simulink model "qdr_vacc_10"  (Simulink 7.9)
settings: Solver=ode45  StartTime=0.0  StopTime=10.0  RelTol=1e-3
libraries: xbsIndex_r4 x8, casper_library_accumulators x1
settings Model: Creator=tfiliba  LastModifiedBy=tfiliba

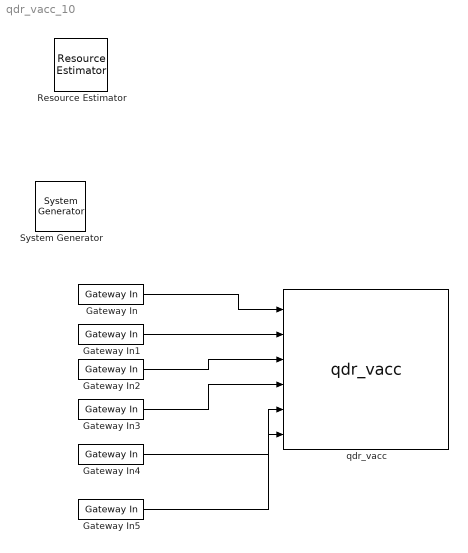
== system qdr_vacc_10 ==
  " System Generator" : xbsIndex_r4/ System Generator  Tag=genX  xilinxfamily=Kintex7  part=xc7k325t  speed=-3  package=fbg676  synthesis_tool=XST  clock_wrapper=Clock Enables  directory=./netlist  proj_type=Project Navigator  Synth_file=XST Defaults  Impl_file=ISE Defaults  testbench=off  simulink_period=1  sysclk_period=10  dcm_input_clock_period=10  incr_netlist=off  trim_vbits=Everywhere in SubSystem  dbl_ovrd=According to Block Masks  core_generation=According to Block Masks  run_coregen=off  deprecated_control=off  eval_field=0  block_type=sysgen
  Gateway In : xbsIndex_r4/Gateway In  gui_display_data_type=Fixed-point  arith_type="Signed  (2's comp)"  n_bits=16  bin_pt=14  preci_type=Single  exp_width=8  frac_width=24  quantization="Round  (unbiased: +/- Inf)"  overflow=Saturate  period=1  dbl_ovrd=off  timing_constraint=None  locs_specified=off  LOCs={}  UseAsADC=off  ADCChannel='1'  inherit_from_input=off  hdl_port=on  block_type=gatewayin
      settings: xl_area=[0 0 0 0 16 0 0]
  Gateway In1 : xbsIndex_r4/Gateway In  gui_display_data_type=Boolean  arith_type=Boolean  n_bits=16  bin_pt=14  preci_type=Single  exp_width=8  frac_width=24  quantization="Round  (unbiased: +/- Inf)"  overflow=Saturate  period=1  dbl_ovrd=off  timing_constraint=None  locs_specified=off  LOCs={}  UseAsADC=off  ADCChannel='1'  inherit_from_input=off  hdl_port=on  block_type=gatewayin
      settings: xl_area=[0 0 0 0 1 0 0]
  Gateway In2 : xbsIndex_r4/Gateway In  gui_display_data_type=Fixed-point  arith_type="Signed  (2's comp)"  n_bits=32  bin_pt=0  preci_type=Single  exp_width=8  frac_width=24  quantization="Round  (unbiased: +/- Inf)"  overflow=Saturate  period=1  dbl_ovrd=off  timing_constraint=None  locs_specified=off  LOCs={}  UseAsADC=off  ADCChannel='1'  inherit_from_input=off  hdl_port=on  block_type=gatewayin
      settings: xl_area=[0 0 0 0 32 0 0]
  Gateway In3 : xbsIndex_r4/Gateway In  gui_display_data_type=Fixed-point  arith_type=Unsigned  n_bits=4  bin_pt=0  preci_type=Single  exp_width=8  frac_width=24  quantization="Round  (unbiased: +/- Inf)"  overflow=Saturate  period=1  dbl_ovrd=off  timing_constraint=None  locs_specified=off  LOCs={}  UseAsADC=off  ADCChannel='1'  inherit_from_input=off  hdl_port=on  block_type=gatewayin
      settings: xl_area=[0 0 0 0 4 0 0]
  Gateway In4 : xbsIndex_r4/Gateway In  gui_display_data_type=Boolean  arith_type=Boolean  n_bits=16  bin_pt=14  preci_type=Single  exp_width=8  frac_width=24  quantization="Round  (unbiased: +/- Inf)"  overflow=Saturate  period=1  dbl_ovrd=off  timing_constraint=None  locs_specified=off  LOCs={}  UseAsADC=off  ADCChannel='1'  inherit_from_input=off  hdl_port=on  block_type=gatewayin
      settings: xl_area=[0 0 0 0 1 0 0]
  Gateway In5 : xbsIndex_r4/Gateway In  gui_display_data_type=Boolean  arith_type=Boolean  n_bits=16  bin_pt=14  preci_type=Single  exp_width=8  frac_width=24  quantization="Round  (unbiased: +/- Inf)"  overflow=Saturate  period=1  dbl_ovrd=off  timing_constraint=None  locs_specified=off  LOCs={}  UseAsADC=off  ADCChannel='1'  inherit_from_input=off  hdl_port=on  block_type=gatewayin
      settings: xl_area=[0 0 0 0 1 0 0]
  Resource Estimator : xbsIndex_r4/Resource Estimator  Tag=resEstTag  Slices=0  FFs=0  BRAMs=0  LUTs=0  IOBs=0  EBMs=0  TBUFs=0  xl_use_estimator_area=off  est_options=Estimate  xl_estimator_area=[824 828 19 1221 232 0 0]  block_type=resource_estimator
      settings: AttributesFormatString=Resource\nEstimator
  qdr_vacc : casper_library_accumulators/qdr_vacc  vector_len=1024
      link override acc_ctrl/rd_addr/convert: arith_type=Unsigned  n_bits=32  bin_pt=0
      link override qdr/convert_be: n_bits=4
      link override qdr/convert_data_in: n_bits=36
      link override qdr/convert_data_in1: n_bits=36
      link override qdr/qdr_latency: latency=10
      link override qdr/qdr_vacc_10_qdr_vacc_qdr_data_out: n_bits=36
      link override status/convert: arith_type=Unsigned  n_bits=32  bin_pt=0
      settings: AttributesFormatString=Vector Length: 1024
      link override Convert1: xl_area=[0 0 0 0 0 0 0]
      link override Delay2: xl_area=[1 1 0 1 0 0 0]
      link override Delay3: xl_area=[1 1 0 1 0 0 0]
      link override Gateway Out1: xl_area=[0 0 0 0 0 0 0]
      link override Gateway Out10: xl_area=[0 0 0 0 0 0 0]
      link override Gateway Out11: xl_area=[0 0 0 0 0 0 0]
      link override Gateway Out12: xl_area=[0 0 0 0 0 0 0]
      link override Gateway Out13: xl_area=[0 0 0 0 0 0 0]
      link override Gateway Out14: xl_area=[0 0 0 0 0 0 0]
      link override Gateway Out15: xl_area=[0 0 0 0 0 0 0]
      link override Gateway Out16: xl_area=[0 0 0 0 0 0 0]
      link override Gateway Out17: xl_area=[0 0 0 0 0 0 0]
      link override Gateway Out18: xl_area=[0 0 0 0 0 0 0]
      link override Gateway Out19: xl_area=[0 0 0 0 0 0 0]
      link override Gateway Out2: xl_area=[0 0 0 0 0 0 0]
      link override Gateway Out20: xl_area=[0 0 0 0 0 0 0]
      link override Gateway Out21: xl_area=[0 0 0 0 0 0 0]
      link override Gateway Out22: xl_area=[0 0 0 0 0 0 0]
      link override Gateway Out23: xl_area=[0 0 0 0 0 0 0]
      link override Gateway Out24: xl_area=[0 0 0 0 0 0 0]
      link override Gateway Out25: xl_area=[0 0 0 0 0 0 0]
      link override Gateway Out26: xl_area=[0 0 0 0 0 0 0]
      link override Gateway Out27: xl_area=[0 0 0 0 0 0 0]
      link override Gateway Out28: xl_area=[0 0 0 0 0 0 0]
      link override Gateway Out29: xl_area=[0 0 0 0 0 0 0]
      link override Gateway Out3: xl_area=[0 0 0 0 0 0 0]
      link override Gateway Out30: xl_area=[0 0 0 0 0 0 0]
      link override Gateway Out31: xl_area=[0 0 0 0 0 0 0]
      link override Gateway Out32: xl_area=[0 0 0 0 0 0 0]
      link override Gateway Out33: xl_area=[0 0 0 0 0 0 0]
      link override Gateway Out4: xl_area=[0 0 0 0 0 0 0]
      link override Gateway Out5: xl_area=[0 0 0 0 0 0 0]
      link override Gateway Out6: xl_area=[0 0 0 0 0 0 0]
      link override Gateway Out7: xl_area=[0 0 0 0 0 0 0]
      link override Gateway Out8: xl_area=[0 0 0 0 0 0 0]
      link override Gateway Out9: xl_area=[0 0 0 0 0 0 0]
      link override Inverter: xl_area=[0 0 0 0 0 0 0]
      link override Inverter1: xl_area=[0 0 0 0 0 0 0]
      link override Logical1: xl_area=[1 1 0 1 0 0 0]
      link override Logical2: xl_area=[1 0 0 1 0 0 0]
      link override Logical3: xl_area=[1 0 0 1 0 0 0]
      link override Logical4: xl_area=[1 0 0 1 0 0 0]
      link override Logical5: xl_area=[1 0 0 1 0 0 0]
      link override Logical6: xl_area=[1 0 0 1 0 0 0]
      link override Relational: xl_area=[6 0 0 11 0 0 0]
      link override Relational1: xl_area=[3 0 0 5 0 0 0]
      link override acc/AddSub4: xl_area=[4 4 0 4 0 0 0]
      link override acc/AddSub5: xl_area=[32 32 0 32 0 0 0]
      link override acc/rd_addr_sel: xl_area=[18 0 0 36 0 0 0]
      link override acc_ctrl/Delay1: xl_area=[1 1 0 0 0 0 0]
      link override acc_ctrl/Delay2: xl_area=[1 1 0 1 0 0 0]
      link override acc_ctrl/Delay3: xl_area=[1 1 0 1 0 0 0]
      link override acc_ctrl/Delay4: xl_area=[5 10 0 0 0 0 0]
      link override acc_ctrl/Delay6: xl_area=[1 1 0 0 0 0 0]
      link override acc_ctrl/Gateway Out1: xl_area=[0 0 0 0 0 0 0]
      link override acc_ctrl/Gateway Out10: xl_area=[0 0 0 0 0 0 0]
      link override acc_ctrl/Gateway Out11: xl_area=[0 0 0 0 0 0 0]
      link override acc_ctrl/Gateway Out12: xl_area=[0 0 0 0 0 0 0]
      link override acc_ctrl/Gateway Out13: xl_area=[0 0 0 0 0 0 0]
      link override acc_ctrl/Gateway Out14: xl_area=[0 0 0 0 0 0 0]
      link override acc_ctrl/Gateway Out15: xl_area=[0 0 0 0 0 0 0]
      link override acc_ctrl/Gateway Out16: xl_area=[0 0 0 0 0 0 0]
      link override acc_ctrl/Gateway Out17: xl_area=[0 0 0 0 0 0 0]
      link override acc_ctrl/Gateway Out19: xl_area=[0 0 0 0 0 0 0]
      link override acc_ctrl/Gateway Out2: xl_area=[0 0 0 0 0 0 0]
      link override acc_ctrl/Gateway Out22: xl_area=[0 0 0 0 0 0 0]
      link override acc_ctrl/Gateway Out28: xl_area=[0 0 0 0 0 0 0]
      link override acc_ctrl/Gateway Out3: xl_area=[0 0 0 0 0 0 0]
      link override acc_ctrl/Gateway Out4: xl_area=[0 0 0 0 0 0 0]
      link override acc_ctrl/Gateway Out5: xl_area=[0 0 0 0 0 0 0]
      link override acc_ctrl/Gateway Out6: xl_area=[0 0 0 0 0 0 0]
      link override acc_ctrl/Gateway Out7: xl_area=[0 0 0 0 0 0 0]
      link override acc_ctrl/Gateway Out8: xl_area=[0 0 0 0 0 0 0]
      link override acc_ctrl/Gateway Out9: xl_area=[0 0 0 0 0 0 0]
      link override acc_ctrl/Inverter: xl_area=[0 0 0 0 0 0 0]
      link override acc_ctrl/Inverter1: xl_area=[0 0 0 0 0 0 0]
      link override acc_ctrl/Inverter2: xl_area=[0 0 0 0 0 0 0]
      link override acc_ctrl/Inverter3: xl_area=[0 0 0 0 0 0 0]
      link override acc_ctrl/Inverter4: xl_area=[0 0 0 0 0 0 0]
      link override acc_ctrl/Inverter5: xl_area=[0 0 0 0 0 0 0]
      link override acc_ctrl/Inverter6: xl_area=[0 0 0 0 0 0 0]
      link override acc_ctrl/Inverter7: xl_area=[0 0 0 0 0 0 0]
      link override acc_ctrl/Inverter8: xl_area=[0 0 0 0 0 0 0]
      link override acc_ctrl/Logical1: xl_area=[1 0 0 1 0 0 0]
      link override acc_ctrl/Logical10: xl_area=[1 0 0 1 0 0 0]
      link override acc_ctrl/Logical11: xl_area=[1 0 0 1 0 0 0]
      link override acc_ctrl/Logical2: xl_area=[1 0 0 1 0 0 0]
      link override acc_ctrl/Logical3: xl_area=[1 0 0 1 0 0 0]
      link override acc_ctrl/Logical4: xl_area=[1 0 0 1 0 0 0]
      link override acc_ctrl/Logical5: xl_area=[1 0 0 1 0 0 0]
      link override acc_ctrl/Logical6: xl_area=[1 0 0 1 0 0 0]
      link override acc_ctrl/Logical7: xl_area=[1 0 0 1 0 0 0]
      link override acc_ctrl/Logical8: xl_area=[1 0 0 1 0 0 0]
      link override acc_ctrl/Logical9: xl_area=[1 0 0 1 0 0 0]
      link override acc_ctrl/Register1: xl_area=[1 1 0 0 0 0 0]
      link override acc_ctrl/Register4: xl_area=[1 1 0 0 0 0 0]
      link override acc_ctrl/Relational: xl_area=[6 0 0 11 0 0 0]
      link override acc_ctrl/Relational2: xl_area=[24 0 0 47 0 0 0]
      link override acc_ctrl/Relational3: xl_area=[6 0 0 11 0 0 0]
      link override acc_ctrl/delay_adder: xl_area=[5 10 0 10 0 0 0]
      link override acc_ctrl/delay_blank_qdr: xl_area=[1 1 0 1 0 0 0]
      link override acc_ctrl/delay_even_addr: xl_area=[5 10 0 0 0 0 0]
      link override acc_ctrl/delay_even_addr1: xl_area=[1 1 0 0 0 0 0]
      link override acc_ctrl/delay_even_addr2: xl_area=[1 1 0 0 0 0 0]
      link override acc_ctrl/delay_for_even_op: xl_area=[1 1 0 0 0 0 0]
      link override acc_ctrl/delay_qdr: xl_area=[5 10 0 10 0 0 0]
      link override acc_ctrl/delay_rd_align: xl_area=[1 1 0 1 0 0 0]
      link override acc_ctrl/delay_rd_align1: xl_area=[1 1 0 1 0 0 0]
      link override acc_ctrl/delay_rd_wr_align1: xl_area=[1 1 0 1 0 0 0]
      link override acc_ctrl/delay_wr_align: xl_area=[5 10 0 10 0 0 0]
      link override acc_ctrl/delay_wr_align1: xl_area=[1 1 0 1 0 0 0]
      link override acc_ctrl/delay_wr_align2: xl_area=[1 1 0 1 0 0 0]
      link override acc_ctrl/delay_wr_align3: xl_area=[1 1 0 1 0 0 0]
      link override acc_ctrl/ease_timing1: xl_area=[8 16 0 0 0 0 0]
      link override acc_ctrl/pulse_ext/Counter3: xl_area=[4 5 0 6 0 0 0]
      link override acc_ctrl/pulse_ext/Gateway Out1: xl_area=[0 0 0 0 0 0 0]
      link override acc_ctrl/pulse_ext/Gateway Out2: xl_area=[0 0 0 0 0 0 0]
      link override acc_ctrl/pulse_ext/Gateway Out3: xl_area=[0 0 0 0 0 0 0]
      link override acc_ctrl/pulse_ext/Gateway Out31: xl_area=[0 0 0 0 0 0 0]
      link override acc_ctrl/pulse_ext/Logical1: xl_area=[1 0 0 1 0 0 0]
      link override acc_ctrl/pulse_ext/Relational5: xl_area=[2 0 0 3 0 0 0]
      link override acc_ctrl/pulse_ext1/Counter3: xl_area=[3 4 0 4 0 0 0]
      link override acc_ctrl/pulse_ext1/Logical: xl_area=[1 0 0 1 0 0 0]
      link override acc_ctrl/pulse_ext1/Logical1: xl_area=[1 0 0 1 0 0 0]
      link override acc_ctrl/pulse_ext1/Register: xl_area=[1 1 0 0 0 0 0]
      link override acc_ctrl/pulse_ext1/Relational5: xl_area=[1 0 0 2 0 0 0]
      link override acc_ctrl/rb_addr: xl_area=[6 10 0 10 0 0 0]
      link override acc_ctrl/rd_addr/convert: xl_area=[0 0 0 0 0 0 0]
      link override acc_ctrl/rd_addr/qdr_vacc_10_qdr_vacc_acc_ctrl_rd_addr_user_data_in: xl_area=[0 0 0 0 32 0 0]
      link override acc_ctrl/rd_addr_cnt: xl_area=[6 10 0 10 0 0 0]
      link override acc_ctrl/rd_addr_sel: xl_area=[5 0 0 10 0 0 0]
      link override acc_ctrl/rd_nwr: xl_area=[5 0 0 10 0 0 0]
      link override acc_ctrl/reg_del: xl_area=[5 10 0 0 0 0 0]
      link override acc_ctrl/vect_cnt: xl_area=[17 32 0 32 0 0 0]
      link override delay: xl_area=[18 36 0 0 0 0 0]
      link override delay1: xl_area=[1 1 0 0 0 0 0]
      link override delay2: xl_area=[1 1 0 0 0 0 0]
      link override fifo_in: xl_area=[29 32 9 50 0 0 0]
      link override fifo_out: xl_area=[29 32 10 50 0 0 0]
      link override make_odd_delay: xl_area=[18 36 0 0 0 0 0]
      link override make_odd_delay1: xl_area=[1 1 0 0 0 0 0]
      link override negedge_delay/Counter3: xl_area=[13 24 0 24 0 0 0]
      link override negedge_delay/Delay: xl_area=[1 1 0 0 0 0 0]
      link override negedge_delay/Logical: xl_area=[1 0 0 1 0 0 0]
      link override negedge_delay/Relational5: xl_area=[13 0 0 25 0 0 0]
      link override negedge_delay/negedge/Delay: xl_area=[1 1 0 0 0 0 0]
      link override negedge_delay/negedge/Inverter: xl_area=[0 0 0 0 0 0 0]
      link override negedge_delay/negedge/Logical: xl_area=[1 0 0 1 0 0 0]
      link override negedge_delay1/Counter3: xl_area=[13 24 0 24 0 0 0]
      link override negedge_delay1/Delay: xl_area=[1 1 0 0 0 0 0]
      link override negedge_delay1/Logical: xl_area=[1 0 0 1 0 0 0]
      link override negedge_delay1/Relational5: xl_area=[13 0 0 25 0 0 0]
      link override negedge_delay1/negedge/Delay: xl_area=[1 1 0 0 0 0 0]
      link override negedge_delay1/negedge/Inverter: xl_area=[0 0 0 0 0 0 0]
      link override negedge_delay1/negedge/Logical: xl_area=[1 0 0 1 0 0 0]
      link override negedge_delay10/Counter3: xl_area=[13 24 0 24 0 0 0]
      link override negedge_delay10/Delay: xl_area=[1 1 0 0 0 0 0]
      link override negedge_delay10/Logical: xl_area=[1 0 0 1 0 0 0]
      link override negedge_delay10/Relational5: xl_area=[13 0 0 25 0 0 0]
      link override negedge_delay10/negedge/Delay: xl_area=[1 1 0 0 0 0 0]
      link override negedge_delay10/negedge/Inverter: xl_area=[0 0 0 0 0 0 0]
      link override negedge_delay10/negedge/Logical: xl_area=[1 0 0 1 0 0 0]
      link override negedge_delay11/Counter3: xl_area=[13 24 0 24 0 0 0]
      link override negedge_delay11/Delay: xl_area=[1 1 0 0 0 0 0]
      link override negedge_delay11/Logical: xl_area=[1 0 0 1 0 0 0]
      link override negedge_delay11/Relational5: xl_area=[13 0 0 25 0 0 0]
      link override negedge_delay11/negedge/Delay: xl_area=[1 1 0 0 0 0 0]
      link override negedge_delay11/negedge/Inverter: xl_area=[0 0 0 0 0 0 0]
      link override negedge_delay11/negedge/Logical: xl_area=[1 0 0 1 0 0 0]
      link override negedge_delay12/Counter3: xl_area=[13 24 0 24 0 0 0]
      link override negedge_delay12/Delay: xl_area=[1 1 0 0 0 0 0]
      link override negedge_delay12/Logical: xl_area=[1 0 0 1 0 0 0]
      link override negedge_delay12/Relational5: xl_area=[13 0 0 25 0 0 0]
      link override negedge_delay12/negedge/Delay: xl_area=[1 1 0 0 0 0 0]
      link override negedge_delay12/negedge/Inverter: xl_area=[0 0 0 0 0 0 0]
      link override negedge_delay12/negedge/Logical: xl_area=[1 0 0 1 0 0 0]
      link override negedge_delay13/Counter3: xl_area=[13 24 0 24 0 0 0]
      link override negedge_delay13/Delay: xl_area=[1 1 0 0 0 0 0]
      link override negedge_delay13/Logical: xl_area=[1 0 0 1 0 0 0]
      link override negedge_delay13/Relational5: xl_area=[13 0 0 25 0 0 0]
      link override negedge_delay13/negedge/Delay: xl_area=[1 1 0 0 0 0 0]
      link override negedge_delay13/negedge/Inverter: xl_area=[0 0 0 0 0 0 0]
      link override negedge_delay13/negedge/Logical: xl_area=[1 0 0 1 0 0 0]
      link override negedge_delay2/Counter3: xl_area=[13 24 0 24 0 0 0]
      link override negedge_delay2/Delay: xl_area=[1 1 0 0 0 0 0]
      link override negedge_delay2/Logical: xl_area=[1 0 0 1 0 0 0]
      link override negedge_delay2/Relational5: xl_area=[13 0 0 25 0 0 0]
      link override negedge_delay2/negedge/Delay: xl_area=[1 1 0 0 0 0 0]
      link override negedge_delay2/negedge/Inverter: xl_area=[0 0 0 0 0 0 0]
      link override negedge_delay2/negedge/Logical: xl_area=[1 0 0 1 0 0 0]
      link override negedge_delay3/Counter3: xl_area=[13 24 0 24 0 0 0]
      link override negedge_delay3/Delay: xl_area=[1 1 0 0 0 0 0]
      link override negedge_delay3/Logical: xl_area=[1 0 0 1 0 0 0]
      link override negedge_delay3/Relational5: xl_area=[13 0 0 25 0 0 0]
      link override negedge_delay3/negedge/Delay: xl_area=[1 1 0 0 0 0 0]
      link override negedge_delay3/negedge/Inverter: xl_area=[0 0 0 0 0 0 0]
      link override negedge_delay3/negedge/Logical: xl_area=[1 0 0 1 0 0 0]
      link override negedge_delay4/Counter3: xl_area=[13 24 0 24 0 0 0]
      link override negedge_delay4/Delay: xl_area=[1 1 0 0 0 0 0]
      link override negedge_delay4/Logical: xl_area=[1 0 0 1 0 0 0]
      link override negedge_delay4/Relational5: xl_area=[13 0 0 25 0 0 0]
      link override negedge_delay4/negedge/Delay: xl_area=[1 1 0 0 0 0 0]
      link override negedge_delay4/negedge/Inverter: xl_area=[0 0 0 0 0 0 0]
      link override negedge_delay4/negedge/Logical: xl_area=[1 0 0 1 0 0 0]
      link override negedge_delay5/Counter3: xl_area=[13 24 0 24 0 0 0]
      link override negedge_delay5/Delay: xl_area=[1 1 0 0 0 0 0]
      link override negedge_delay5/Logical: xl_area=[1 0 0 1 0 0 0]
      link override negedge_delay5/Relational5: xl_area=[13 0 0 25 0 0 0]
      link override negedge_delay5/negedge/Delay: xl_area=[1 1 0 0 0 0 0]
      link override negedge_delay5/negedge/Inverter: xl_area=[0 0 0 0 0 0 0]
      link override negedge_delay5/negedge/Logical: xl_area=[1 0 0 1 0 0 0]
      link override negedge_delay6/Counter3: xl_area=[13 24 0 24 0 0 0]
      link override negedge_delay6/Delay: xl_area=[1 1 0 0 0 0 0]
      link override negedge_delay6/Logical: xl_area=[1 0 0 1 0 0 0]
      link override negedge_delay6/Relational5: xl_area=[13 0 0 25 0 0 0]
      link override negedge_delay6/negedge/Delay: xl_area=[1 1 0 0 0 0 0]
      link override negedge_delay6/negedge/Inverter: xl_area=[0 0 0 0 0 0 0]
      link override negedge_delay6/negedge/Logical: xl_area=[1 0 0 1 0 0 0]
      link override negedge_delay7/Counter3: xl_area=[13 24 0 24 0 0 0]
      link override negedge_delay7/Delay: xl_area=[1 1 0 0 0 0 0]
      link override negedge_delay7/Logical: xl_area=[1 0 0 1 0 0 0]
      link override negedge_delay7/Relational5: xl_area=[13 0 0 25 0 0 0]
      link override negedge_delay7/negedge/Delay: xl_area=[1 1 0 0 0 0 0]
      link override negedge_delay7/negedge/Inverter: xl_area=[0 0 0 0 0 0 0]
      link override negedge_delay7/negedge/Logical: xl_area=[1 0 0 1 0 0 0]
      link override negedge_delay8/Counter3: xl_area=[13 24 0 24 0 0 0]
      link override negedge_delay8/Delay: xl_area=[1 1 0 0 0 0 0]
      link override negedge_delay8/Logical: xl_area=[1 0 0 1 0 0 0]
      link override negedge_delay8/Relational5: xl_area=[13 0 0 25 0 0 0]
      link override negedge_delay8/negedge/Delay: xl_area=[1 1 0 0 0 0 0]
      link override negedge_delay8/negedge/Inverter: xl_area=[0 0 0 0 0 0 0]
      link override negedge_delay8/negedge/Logical: xl_area=[1 0 0 1 0 0 0]
      link override negedge_delay9/Counter3: xl_area=[13 24 0 24 0 0 0]
      link override negedge_delay9/Delay: xl_area=[1 1 0 0 0 0 0]
      link override negedge_delay9/Logical: xl_area=[1 0 0 1 0 0 0]
      link override negedge_delay9/Relational5: xl_area=[13 0 0 25 0 0 0]
      link override negedge_delay9/negedge/Delay: xl_area=[1 1 0 0 0 0 0]
      link override negedge_delay9/negedge/Inverter: xl_area=[0 0 0 0 0 0 0]
      link override negedge_delay9/negedge/Logical: xl_area=[1 0 0 1 0 0 0]
      link override out_valid_delay: xl_area=[1 1 0 0 0 0 0]
      link override qdr/Delay1: xl_area=[1 1 0 0 0 0 0]
      link override qdr/Inverter2: xl_area=[0 0 0 0 0 0 0]
      link override qdr/Logical: xl_area=[1 0 0 1 0 0 0]
      link override qdr/Logical1: xl_area=[1 0 0 1 0 0 0]
      link override qdr/convert_ack: xl_area=[0 0 0 0 0 0 0]
      link override qdr/convert_address: xl_area=[0 0 0 0 0 0 0]
      link override qdr/convert_be: xl_area=[0 0 0 0 0 0 0]
      link override qdr/convert_cal_fail: xl_area=[0 0 0 0 0 0 0]
      link override qdr/convert_data_in: xl_area=[0 0 0 0 0 0 0]
      link override qdr/convert_data_in1: xl_area=[0 0 0 0 0 0 0]
      link override qdr/convert_rd_en: xl_area=[0 0 0 0 0 0 0]
      link override qdr/convert_ready: xl_area=[0 0 0 0 0 0 0]
      link override qdr/convert_wr_en: xl_area=[0 0 0 0 0 0 0]
      link override qdr/prev_rd: xl_area=[1 1 0 0 0 0 0]
      link override qdr/qdr_latency: xl_area=[1 1 0 1 0 0 0]
      link override qdr/qdr_vacc_10_qdr_vacc_qdr_ack: xl_area=[0 0 0 0 1 0 0]
      link override qdr/qdr_vacc_10_qdr_vacc_qdr_address: xl_area=[0 0 0 0 32 0 0]
      link override qdr/qdr_vacc_10_qdr_vacc_qdr_be: xl_area=[0 0 0 0 4 0 0]
      link override qdr/qdr_vacc_10_qdr_vacc_qdr_cal_fail: xl_area=[0 0 0 0 1 0 0]
      link override qdr/qdr_vacc_10_qdr_vacc_qdr_data_in: xl_area=[0 0 0 0 36 0 0]
      link override qdr/qdr_vacc_10_qdr_vacc_qdr_data_out: xl_area=[0 0 0 0 36 0 0]
      link override qdr/qdr_vacc_10_qdr_vacc_qdr_phy_ready: xl_area=[0 0 0 0 1 0 0]
      link override qdr/qdr_vacc_10_qdr_vacc_qdr_rd_en: xl_area=[0 0 0 0 1 0 0]
      link override qdr/qdr_vacc_10_qdr_vacc_qdr_wr_en: xl_area=[0 0 0 0 1 0 0]
      link override qdr_del_comp: xl_area=[5 10 0 10 0 0 0]
      link override qdr_del_comp1: xl_area=[1 1 0 1 0 0 0]
      link override qdr_del_comp2: xl_area=[18 36 0 36 0 0 0]
      link override qdr_del_comp3: xl_area=[18 36 0 36 0 0 0]
      link override qdr_del_comp4: xl_area=[1 1 0 1 0 0 0]
      link override qdr_del_comp5: xl_area=[1 1 0 1 0 0 0]
      link override qdr_del_comp6: xl_area=[1 1 0 1 0 0 0]
      link override qdr_del_comp7: xl_area=[1 1 0 1 0 0 0]
      link override qdr_del_comp8: xl_area=[1 1 0 1 0 0 0]
      link override rst_delay: xl_area=[1 1 0 1 0 0 0]
      link override stat_del: xl_area=[7 14 0 0 0 0 0]
      link override stat_del1: xl_area=[1 1 0 0 0 0 0]
      link override stat_del10: xl_area=[1 1 0 0 0 0 0]
      link override stat_del11: xl_area=[1 1 0 0 0 0 0]
      link override stat_del12: xl_area=[1 1 0 0 0 0 0]
      link override stat_del13: xl_area=[1 1 0 0 0 0 0]
      link override stat_del14: xl_area=[1 1 0 0 0 0 0]
      link override stat_del15: xl_area=[1 1 0 0 0 0 0]
      link override stat_del2: xl_area=[1 1 0 0 0 0 0]
      link override stat_del3: xl_area=[1 1 0 0 0 0 0]
      link override stat_del4: xl_area=[1 1 0 0 0 0 0]
      link override stat_del5: xl_area=[1 1 0 0 0 0 0]
      link override stat_del6: xl_area=[1 1 0 0 0 0 0]
      link override stat_del7: xl_area=[1 1 0 0 0 0 0]
      link override stat_del8: xl_area=[1 1 0 0 0 0 0]
      link override stat_del9: xl_area=[1 1 0 0 0 0 0]
      link override status/convert: xl_area=[0 0 0 0 0 0 0]
      link override status/qdr_vacc_10_qdr_vacc_status_user_data_in: xl_area=[0 0 0 0 32 0 0]
      link override sync_count: xl_area=[6 10 0 10 0 0 0]
  wires:
  Gateway In/1 -> qdr_vacc/1
  Gateway In1/1 -> qdr_vacc/2
  Gateway In2/1 -> qdr_vacc/3
  Gateway In3/1 -> qdr_vacc/4
  Gateway In4/1 -> qdr_vacc/5
  Gateway In5/1 -> qdr_vacc/6
